simulink model "JFK_Sleep_I"  (R2015a)
settings: Solver=ode3  StartTime=0.0  StopTime=3000  FixedStep=0.01  RelTol=1e-5
undefined symbols (not defined in the file): D, H0, Imax, n0, T, x0, xc0
settings Model: Creator=Zhang Jiaxiang  LastModifiedBy=Jiawei Yin
settings DataIOCC: LimitDataPoints=off  SignalLoggingSaveFormat=ModelDataLogs
settings OptimizationCC: ExpressionDepthLimit=2147483647
settings DebuggingCC: UnderspecifiedInitializationDetection=Classic  MergeDetectMultiDrivingBlocksExec=none  FcnCallInpInsideContextMsg=UseLocalSettings  StateNameClashWarn=warning
settings GRTTargetCC: CombineOutputUpdateFcns=off  GRTInterface=on

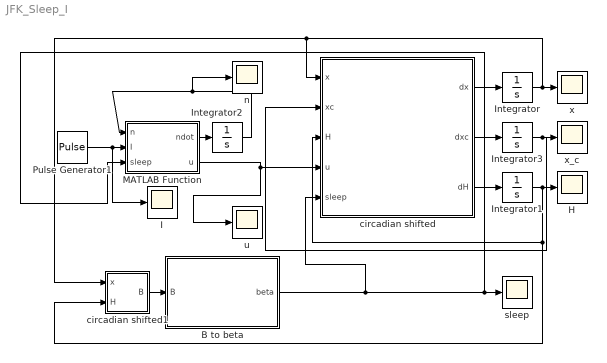
== system JFK_Sleep_I ==
  "B to beta " : Subsystem
  H : Scope
      settings: TimeRange=auto  MaxDataPoints=1000000  SaveName=H  YMin=-0.03001  YMax=0.84118  SampleTime=-1  DataFormat=Array
  I : Scope
      settings: TimeRange=auto  MaxDataPoints=100000000  SaveName=I  YMin=-0.00064  YMax=0.00577  SampleTime=-1  DataFormat=Array
  Integrator : Integrator  InitialCondition=x0
  Integrator1 : Integrator  InitialCondition=H0
  Integrator2 : Integrator  InitialCondition=n0
  Integrator3 : Integrator  InitialCondition=xc0
  MATLAB Function : MATLAB Function  TreatAsAtomicUnit=on
      settings: PermitHierarchicalResolution=ParametersOnly
  Pulse Generator1 : DiscretePulseGenerator  PulseType=Time based  Amplitude=Imax  Period=T  PulseWidth=D
  circadian shifted : MATLAB Function  TreatAsAtomicUnit=on
      settings: PermitHierarchicalResolution=ParametersOnly
  circadian shifted1 : MATLAB Function  TreatAsAtomicUnit=on
      settings: PermitHierarchicalResolution=ParametersOnly
  n : Scope
      settings: TimeRange=auto  MaxDataPoints=1000000  SaveName=n  YMin=-0.03001  YMax=0.84118  SampleTime=-1  DataFormat=Array
  sleep : Scope
      settings: TimeRange=auto  MaxDataPoints=100000000  SaveName=sleep  YMin=-0.125  YMax=1.125  SampleTime=-1  DataFormat=Array
  u : Scope
      settings: TimeRange=auto  MaxDataPoints=1000000  SaveName=u  YMin=-0.03001  YMax=0.84118  SampleTime=-1  DataFormat=Array
  x : Scope
      settings: TimeRange=auto  MaxDataPoints=1000000  SaveName=x  YMin=-0.78539  YMax=7.06847  SampleTime=-1  DataFormat=Array
  x_c : Scope
      settings: TimeRange=auto  MaxDataPoints=1000000  SaveName=xc  YMin=-0.78539  YMax=7.06847  SampleTime=-1  DataFormat=Array
  wires:
  circadian shifted/1(dx) -> Integrator/1
  circadian shifted/3(dH) -> Integrator1/1
  Integrator1/1 -> circadian shifted/3(H), circadian shifted1/2(H), H/1
  MATLAB Function/1(ndot) -> Integrator2/1
  Pulse Generator1/1 -> I/1, MATLAB Function/2(I)
  Integrator2/1 -> n/1, MATLAB Function/1(n)
  MATLAB Function/2(u) -> u/1, circadian shifted/4(u)
  circadian shifted1/1(B) -> "B to beta "/1(B)
  "B to beta "/1(beta) -> circadian shifted/5(sleep), MATLAB Function/3(sleep), sleep/1
  Integrator/1 -> x/1, circadian shifted1/1(x), circadian shifted/1(x)
  circadian shifted/2(dxc) -> Integrator3/1
  Integrator3/1 -> circadian shifted/2(xc), x_c/1

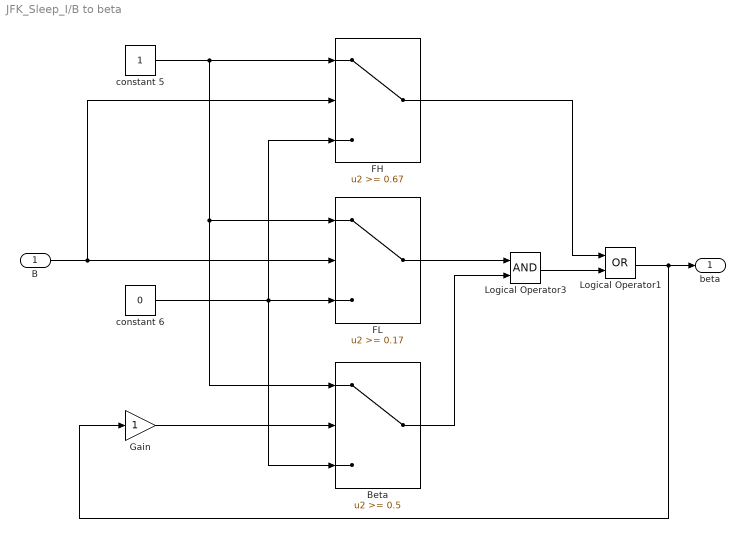
== system JFK_Sleep_I/B to beta  ==
  B : Inport
  Beta : Switch  Threshold=0.5
  FH : Switch  Threshold=0.67
  FL : Switch  Threshold=0.17
  Gain : Gain
  Logical Operator1 : Logic  Operator=OR  AllPortsSameDT=off  OutDataTypeStr=boolean
  Logical Operator3 : Logic  AllPortsSameDT=off  OutDataTypeStr=boolean
  constant 5 : Constant
  constant 6 : Constant  Value=0
  beta : Outport
  wires:
  constant 5/1 -> Beta/1, FL/1, FH/1
  constant 6/1 -> Beta/3, FH/3, FL/3
  B/1 -> FH/2, FL/2
  Logical Operator1/1 -> Gain/1, beta/1
  Gain/1 -> Beta/2
  FL/1 -> Logical Operator3/1
  Beta/1 -> Logical Operator3/2
  Logical Operator3/1 -> Logical Operator1/2
  FH/1 -> Logical Operator1/1

== matlab function JFK_Sleep_I/circadian shifted ==
  data: x input; xc input; H input; u input; dx output; dxc output; dH output; sleep input
function [ dx,dxc,dH] = fcn(x,xc,H,u,sleep)
%#eml
q = 1/3;
taux = 24.2;
k = 0.55;
mu=0.13;

B = u*(1-0.4*x)*(1-0.4*xc);
omega0=2*pi/24.2;
tr=18.2;
td=4.2;


dx = (pi/12)*(xc + B  + mu*(1/3*x + 4/3*x^3 - 256/105*x^7));
dxc = (pi/12)*(q*B *xc - (24/(taux*0.99729))^2*x - k*B*x);
dH=(1-H)*(1-sleep)/tr-H*sleep/td;

== matlab function JFK_Sleep_I/MATLAB Function ==
  data: n input; I input; ndot output; u output; sleep input
function [ndot,u] = fcn(n,I,sleep)
G=33.75;
alpha0=0.05;
beta=0.0075;
I0=9500;
alpha=alpha0*(I*(1-sleep)/I0)^0.5;
u=G*alpha*(1-n);
ndot=60*[alpha*(1-n)-beta*n];

== matlab function JFK_Sleep_I/circadian shifted1 ==
  data: x input; H input; B output
function B = fcn(x,H)
%#eml
B=H-0.1333*x;
